simulink model "PendulumModel"  (R2018a)
settings: Solver=VariableStepAuto  StartTime=0.0  StopTime=10.0  RelTol=1e-3
values from neighbouring files (symbols this model uses):
  g = 10    [SinglePendulum.m]
  l = 1.5    [SinglePendulum.m]
  m = 4    [SinglePendulum.m]
  M = 5    [SinglePendulum.m]
undefined symbols (not defined in the file or in its folder): b, I
libraries: simulink x1
settings Model: Creator=ounen  LastModifiedBy=ounen
settings SolverCC: DecoupledContinuousIntegration=on  MinimalZcImpactIntegration=on

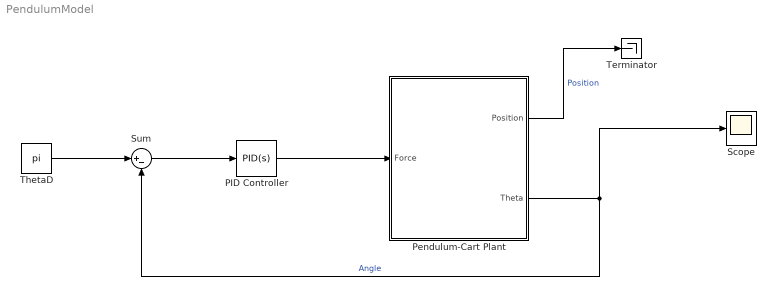
== system PendulumModel ==
  PID Controller : simulink/Continuous/PID Controller  Controller=PID  Form=Parallel  TimeDomain=Continuous-time  SampleTime=-1  IntegratorMethod=Forward Euler  FilterMethod=Forward Euler  ControllerParametersSource=internal  P=15  I=0  D=2.5  UseFilter=on  N=100  TunerSelectOption=Transfer Function Based (PID Tuner App)  InitialConditionSource=internal  InitialConditionForIntegrator=0  InitialConditionForFilter=0  DifferentiatorICPrevScaledInput=0  ExternalReset=none  TrackingMode=off  Kt=1  LimitOutput=off  UpperSaturationLimit=inf  LowerSaturationLimit=-inf  LinearizeAsGain=on  AntiWindupMode=none  Kb=1  POutMin=[]  POutMax=[]  IOutMin=[]  IOutMax=[]  DOutMin=[]  DOutMax=[]  NOutMin=[]  NOutMax=[]  SumOutMin=[]  SumOutMax=[]  SaturationOutMin=[]  SaturationOutMax=[]  PParamMin=[]  PParamMax=[]  IParamMin=[]  IParamMax=[]  DParamMin=[]  DParamMax=[]  NParamMin=[]  NParamMax=[]  KbParamMin=[]  KbParamMax=[]  KtParamMin=[]  KtParamMax=[]  KbOutMin=[]  KbOutMax=[]  KtOutMin=[]  KtOutMax=[]  IntegratorOutMin=[]  IntegratorOutMax=[]  FilterOutMin=[]  FilterOutMax=[]  SumI1OutMin=SumI1OutMin  SumI1OutMax=SumI1OutMax  SumI2OutMin=[]  SumI2OutMax=[]  SumI3OutMin=[]  SumI3OutMax=[]  SumI4OutMin=[]  SumI4OutMax=[]  SumDOutMin=[]  SumDOutMax=[]  DifferentiatorOutMin=[]  DifferentiatorOutMax=[]  FilterDiffOutCoefMin=[]  FilterDiffOutCoefMax=[]  ReciprocalOutMin=[]  ReciprocalOutMax=[]  SumDenOutMin=[]  SumDenOutMax=[]  SumNumOutMin=[]  SumNumOutMax=[]  DivideOutMin=[]  DivideOutMax=[]  IntegratorContinuousStateAttributes=''  IntegratorStateMustResolveToSignalObject=off  IntegratorRTWStateStorageClass=Auto  FilterContinuousStateAttributes=''  FilterStateMustResolveToSignalObject=off  FilterRTWStateStorageClass=Auto  ParallelPVariant=InternalParameters  IdealPVariant=Disabled  IVariant=InternalParameters  DVariant=InternalParameters  IntegratorVariant=Continuous  SatVariant=Disabled  AWVariant=Passthrough  PCopyVariant=Disabled  TRVariant=Disabled  FdbkBlocksVariant=Forward  IdealPFdbkVariant=Disabled  SatFdbkVariant=Disabled  DerivativeFilterVariant=ContFilter  NVariant=InternalParameters  NCopyVariant=Disabled  FilterICVariant=InternalICsFilter  IntegratorICVariant=InternalICs  ExternalResetVariant=Disabled  TRSumVariant=Passthrough
  "Pendulum-Cart Plant " : Subsystem
  Scope : Scope
  Sum : Sum  Inputs=|+-
  Terminator : Terminator
  ThetaD : Constant  Value=pi
  wires:
  "Pendulum-Cart Plant "/2(Theta) -> Scope/1, Sum/2  "Angle"
  PID Controller/1 -> "Pendulum-Cart Plant "/1("Force ")
  ThetaD/1 -> Sum/1
  Sum/1 -> PID Controller/1
  "Pendulum-Cart Plant "/1(Position) -> Terminator/1  "Position"

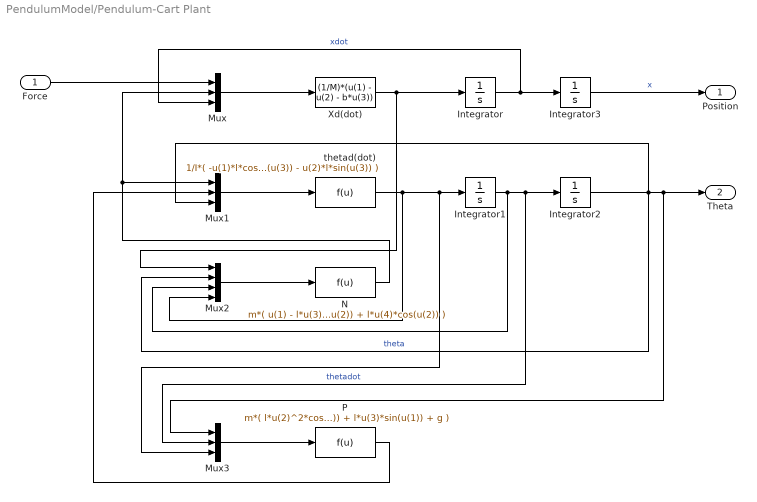
== system PendulumModel/Pendulum-Cart Plant  ==
  "Force " : Inport
  Integrator : Integrator
  Integrator1 : Integrator
  Integrator2 : Integrator  InitialCondition=pi + 0.25  ContinuousStateAttributes='theta'
  Integrator3 : Integrator
  Mux : Mux  Inputs=3
  Mux1 : Mux  Inputs=3
  Mux2 : Mux
  Mux3 : Mux  Inputs=3
  N : Fcn  Expr=m*( u(1) - l*u(3)^2*sin(u(2)) + l*u(4)*cos(u(2)) )
  P : Fcn  Expr=m*( l*u(2)^2*cos(u(1)) + l*u(3)*sin(u(1)) + g )
  Xd(dot) : Fcn  Expr=(1/M)*(u(1) - u(2) - b*u(3))
  thetad(dot) : Fcn  Expr=1/I*( -u(1)*l*cos(u(3)) - u(2)*l*sin(u(3)) )
  Position : Outport
  Theta : Outport  Port=2
  wires:
  N/1 -> Mux1/1, Mux/2
  Integrator2/1 -> Mux2/2, Mux1/3, Theta/1, Mux3/1  "theta"
  Integrator1/1 -> Mux2/3, Mux3/2, Integrator2/1  "thetadot"
  Integrator/1 -> Mux/3, Integrator3/1  "xdot"
  Xd(dot)/1 -> Mux2/1, Integrator/1
  thetad(dot)/1 -> Mux3/3, Integrator1/1, Mux2/4
  Mux/1 -> Xd(dot)/1
  P/1 -> Mux1/2
  Mux3/1 -> P/1
  Mux2/1 -> N/1
  Mux1/1 -> thetad(dot)/1
  "Force "/1 -> Mux/1
  Integrator3/1 -> Position/1  "x"
